simulink library "delay"  (R2019a)
settings: Solver=VariableStepAuto  StartTime=0.0  StopTime=10.0  RelTol=1e-3
settings Model: Creator=Administrator  LastModifiedBy=wangz

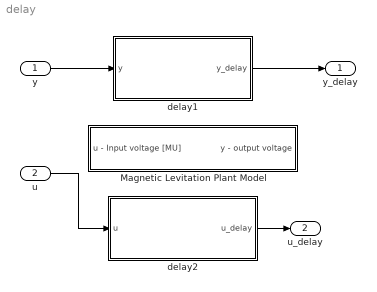
== system delay ==
  "y " : Inport
  "u " : Inport  Port=2
  Magnetic Levitation Plant Model : Subsystem
  "delay1 " : Subsystem
  delay2 : Subsystem
  y_delay : Outport
  "u_delay " : Outport  Port=2
  wires:
  "delay1 "/1(y_delay) -> y_delay/1
  "y "/1 -> "delay1 "/1("y ")
  "u "/1 -> delay2/1("u ")
  delay2/1("u_delay ") -> "u_delay "/1

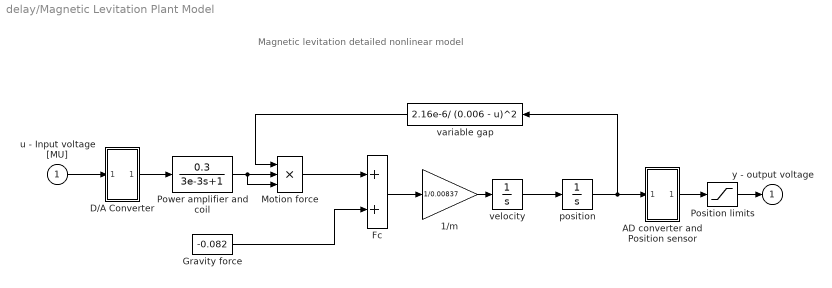
== system delay/Magnetic Levitation Plant Model ==
  note: Magnetic levitation
      | detailed nonlinear model
  u - Input voltage [MU] : Inport
  1/m : Gain  Gain=1/0.00837  SaturateOnIntegerOverflow=on  OutDataTypeStr=Inherit: Same as input  ParamDataTypeStr=Inherit: Same as input
  AD converter and Position sensor : Subsystem
      mask Display: disp('A/D')
  D/A Converter : Subsystem
      mask Display: disp('D/A')
  Fc : Sum  SaturateOnIntegerOverflow=on  InputSameDT=on  OutDataTypeStr=Inherit: Same as first input
  Gravity force : Constant  Value=-0.082
  Motion force : Product  Inputs=3  SaturateOnIntegerOverflow=on  InputSameDT=on  OutDataTypeStr=Inherit: Same as first input
  Position limits : Saturate  UpperLimit=0.998  LowerLimit=0  ZeroCross=off
  Power amplifier and coil : TransferFcn  Numerator=[0.3]  Denominator=[3e-3 1]
  position : Integrator  LimitOutput=on  UpperSaturationLimit=0.005  LowerSaturationLimit=0  ZeroCross=off
  variable gap : Fcn  Expr=2.16e-6/ (0.006 - u)^2
  velocity : Integrator  UpperSaturationLimit=5000000  LowerSaturationLimit=-500000  ZeroCross=off
  y - output voltage : Outport
  wires:
  velocity/1 -> position/1
  variable gap/1 -> Motion force/1
  1/m/1 -> velocity/1
  Fc/1 -> 1/m/1
  Motion force/1 -> Fc/1
  Gravity force/1 -> Fc/2
  D/A Converter/1(out_1) -> Power amplifier and coil/1
  u - Input voltage [MU]/1 -> D/A Converter/1(in_1)
  AD converter and Position sensor/1(out_1) -> Position limits/1
  position/1 -> variable gap/1, AD converter and Position sensor/1(in_1)
  Power amplifier and coil/1 -> Motion force/3, Motion force/2
  Position limits/1 -> y - output voltage/1

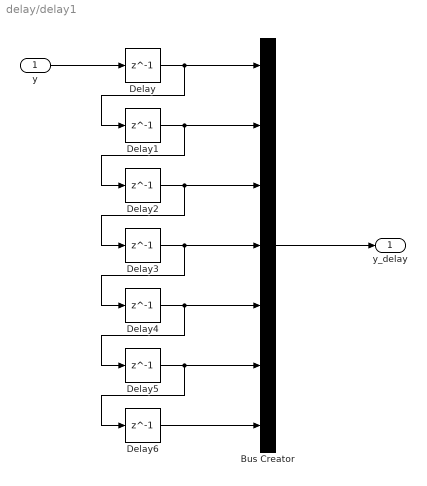
== system delay/delay1  ==
  "y " : Inport
  Bus Creator : BusCreator  Inputs=7
  Delay{,1..6} (7 alike) : Delay  DelayLength=1
  y_delay : Outport
  wires:
  Delay4/1 -> Delay5/1, Bus Creator/5
  "y "/1 -> Delay/1
  Delay6/1 -> Bus Creator/7
  Delay/1 -> Bus Creator/1, Delay1/1
  Delay3/1 -> Bus Creator/4, Delay4/1
  Delay5/1 -> Bus Creator/6, Delay6/1
  Delay1/1 -> Delay2/1, Bus Creator/2
  Delay2/1 -> Bus Creator/3, Delay3/1
  Bus Creator/1 -> y_delay/1

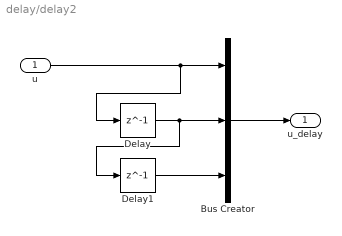
== system delay/delay2 ==
  "u " : Inport
  Bus Creator : BusCreator  Inputs=3
  Delay : Delay  DelayLength=1
  Delay1 : Delay  DelayLength=1
  "u_delay " : Outport
  wires:
  Bus Creator/1 -> "u_delay "/1
  Delay1/1 -> Bus Creator/3
  Delay/1 -> Delay1/1, Bus Creator/2
  "u "/1 -> Delay/1, Bus Creator/1

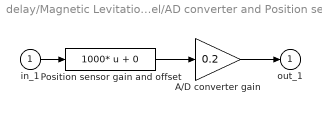
== system delay/Magnetic Levitation Plant Model/AD converter and Position sensor ==
  in_1 : Inport
  A/D converter gain : Gain  Gain=0.2  SaturateOnIntegerOverflow=on  OutDataTypeStr=Inherit: Same as input  ParamDataTypeStr=Inherit: Same as input
  Position sensor gain and offset : Fcn  Expr=1000* u + 0
  out_1 : Outport
  wires:
  in_1/1 -> Position sensor gain and offset/1
  Position sensor gain and offset/1 -> A/D converter gain/1
  A/D converter gain/1 -> out_1/1

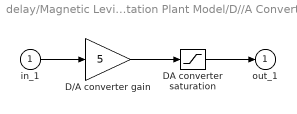
== system delay/Magnetic Levitation Plant Model/D//A Converter ==
  in_1 : Inport
  D/A converter gain : Gain  Gain=5  SaturateOnIntegerOverflow=on  OutDataTypeStr=Inherit: Same as input  ParamDataTypeStr=Inherit: Same as input
  DA converter saturation : Saturate  UpperLimit=5  LowerLimit=-5  ZeroCross=off
  out_1 : Outport
  wires:
  in_1/1 -> D/A converter gain/1
  DA converter saturation/1 -> out_1/1
  D/A converter gain/1 -> DA converter saturation/1
